simulink model "satelitte"  (Simulink 4.00)
settings: Solver=ode45  StartTime=0.0  StopTime=100  FixedStep=0.001  MaxStep=0.001  MinStep=0.00000001  RelTol=1e-3
undefined symbols (not defined in the file): k
settings Model: LastModifiedBy=Gordon

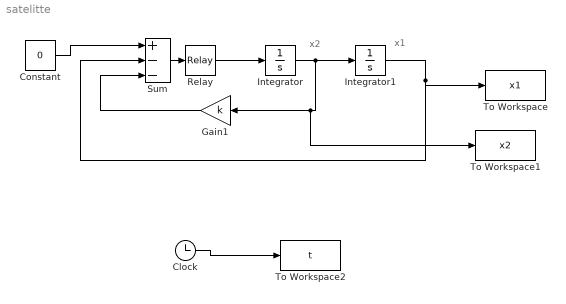
== system satelitte ==
  note: x1
  note: x2
  Clock : Clock
      settings: DisplayTime=off  Decimation=10
  Constant : Constant  Value=0
  Gain1 : Gain  Orientation=left  Gain=k  Multiplication=Element-wise(K.*u)  SaturateOnIntegerOverflow=on
  Integrator : Integrator  ExternalReset=none  InitialConditionSource=internal  InitialCondition=0.0  LimitOutput=off  UpperSaturationLimit=inf  LowerSaturationLimit=-inf  ShowSaturationPort=off  ShowStatePort=off  AbsoluteTolerance=auto
  Integrator1 : Integrator  ExternalReset=none  InitialConditionSource=internal  InitialCondition=-1.0  LimitOutput=off  UpperSaturationLimit=inf  LowerSaturationLimit=-inf  ShowSaturationPort=off  ShowStatePort=off  AbsoluteTolerance=auto
  Relay : Relay  OnSwitchValue=0.001  OffSwitchValue=-0.001  OnOutputValue=1  OffOutputValue=-1
  Sum : Sum  Inputs=+--  SaturateOnIntegerOverflow=on
  To Workspace : ToWorkspace  VariableName=x1  SampleTime=-1  SaveFormat=Array
  To Workspace1 : ToWorkspace  VariableName=x2  SampleTime=-1  SaveFormat=Array
  To Workspace2 : ToWorkspace  VariableName=t  SampleTime=-1  SaveFormat=Array
  wires:
  Sum/1 -> Relay/1
  Integrator/1 -> Integrator1/1, Gain1/1, To Workspace1/1
  Gain1/1 -> Sum/3
  Clock/1 -> To Workspace2/1
  Constant/1 -> Sum/1
  Integrator1/1 -> To Workspace/1, Sum/2
  Relay/1 -> Integrator/1
